simulink model "lab7task"  (R2022b)
settings: Solver=ode45  StartTime=0.0  StopTime=sim_time  RelTol=1e-07  AbsTol=1e-07
values from neighbouring files (symbols this model uses):
  a = 6371+2000    (= 8371)    [lab7taskm.m]
  A0 = [1 0 0; 0 1 0; 0 0 1]    [lab7task1m.m]    (also in lab7taskm.m)
  area = [.06 .06 .04 .06 .06 .04 .12 .12 .12 .12]    [lab7taskm.m]
  C_D = 0.2    [lab7taskm.m]
  density = 0    [lab7taskm.m]
  e = 0.1    [lab7taskm.m]
  eps_Sun = deg2rad(23.45)    [lab7taskm.m]
  euler312_0 = [-atan2(A0(2,1),A0(2,2)); asin(A0(2,3)); -atan2(A0(1,3),A0(3,3))]    [lab7task1m.m]    (also in lab7taskm.m)
  euler313_0 = [-atan2(A0(3,1),A0(3,2)); asin(A0(3,3)); atan2(A0(1,3),A0(2,3))]    [lab7task1m.m]    (also in lab7taskm.m)
  gamma0 = [0;0;1]    [lab7task1m.m]    (also in lab7taskm.m)
  H0 = sqrt((-29615e-9)^2+(-1728e-9)^2+(5186e-9)^2)    [lab7taskm.m]
  I = diag(I)    [lab7task1m.m]    (also in lab7taskm.m)
  I_inv = pinv(I)    [lab7task1m.m]    (also in lab7taskm.m)
  incli = deg2rad(10)    [lab7taskm.m]
  Ir = 0.005    [lab7task1m.m]    (also in lab7taskm.m)
  k = [0;0;1]    [lab7task1m.m]    (also in lab7taskm.m)
  M = [0;0;0]    [lab7task1m.m]    (also in lab7taskm.m)
  m_par = [0.01;0.05;0.01]    [lab7taskm.m]
  mag_tilt = deg2rad(11.5)    [lab7taskm.m]
  Mr = 0    [lab7task1m.m]    (also in lab7taskm.m)
  mu_E = 398600    [lab7task1m.m]    (also in lab7taskm.m = 398600.4418)
  n = sqrt(mu_E/(height+R_E)^3)    [lab7task1m.m]    (also in lab7taskm.m = sqrt(mu_E/a^3))
  n_Sun = sqrt(132712440017.987/R_Sun^3)    [lab7taskm.m]
  Normals = zeros(3,10)    [lab7taskm.m]
  nsurfs = 10    [lab7taskm.m]
  pos = pos-pos_CG    [lab7taskm.m]
  q0 = zeros(4,1)    [lab7task1m.m]    (also in lab7taskm.m)
  R_equat = 6371    [lab7taskm.m]
  R_Sun = 149597870.691    [lab7taskm.m]
  radpressure = radiation/(3e8)    (= 4.52666666667e-06)    [lab7taskm.m]
  rho_d = [.1 .1 .1 .1 .1 .1 .1 .1 .1 .1]    [lab7taskm.m]
  rho_s = [.5 .5 .5 .5 .5 .5 .5 .5 .5 .5]    [lab7taskm.m]
  theta0 = 0    [lab7taskm.m]
  w0 = cat(1,w0,wr0)    [lab7task1m.m]    (also in lab7taskm.m)
  w_E = 2*pi/(23*3600+56*60+4.09)    (= 7.29211590023e-05)    [lab7taskm.m]
libraries: matrix_library x7, vrlib x5
settings Model: Creator=a1pab  LastModifiedBy=a1pab

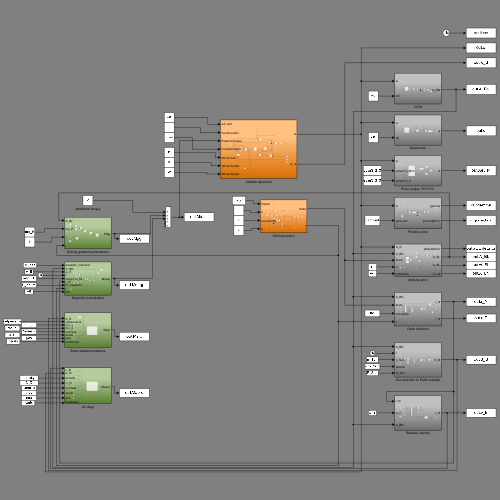
[thumbnail: Simulink's stored preview of the top-level diagram]
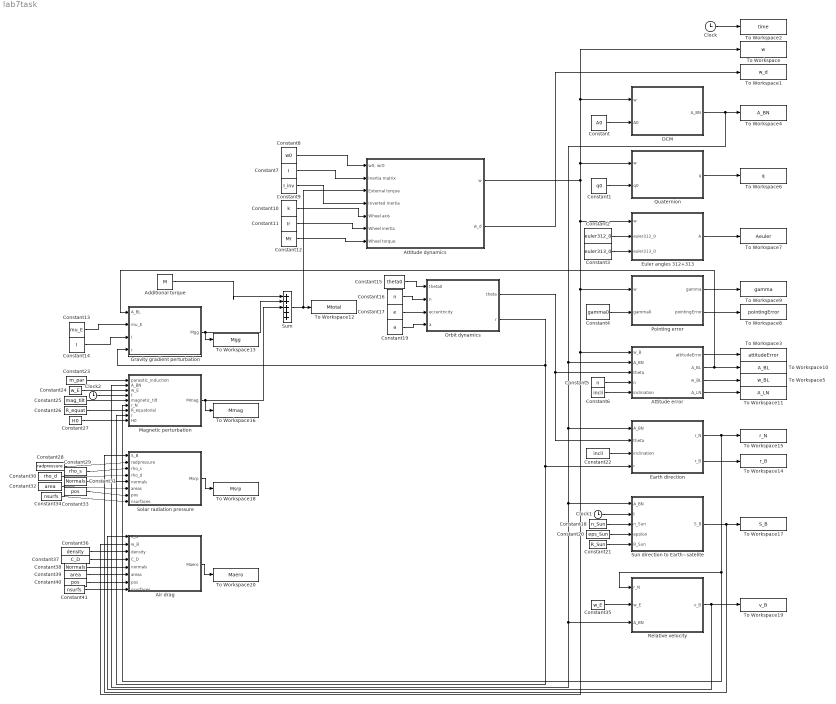
== system lab7task ==
  Additional torque : Constant  Value=M  VectorParams1D=off
  Air drag : Subsystem
  Attitude dynamics : Subsystem
  Attitude error : Subsystem
  Clock : Clock
  Clock1 : Clock
  Clock2 : Clock
  Constant : Constant  Value=A0  VectorParams1D=off
  Constant1 : Constant  Value=q0  VectorParams1D=off
  Constant10 : Constant  Value=k  VectorParams1D=off
  Constant11 : Constant  Value=Ir
  Constant12 : Constant  Value=Mr
  Constant13 : Constant  Value=mu_E
  Constant14 : Constant  Value=I  VectorParams1D=off
  Constant15 : Constant  Value=theta0
  Constant16 : Constant  Value=n
  Constant17 : Constant  Value=e
  Constant18 : Constant  Value=n_Sun
  Constant19 : Constant  Value=a
  Constant2 : Constant  Value=euler312_0  VectorParams1D=off
  Constant20 : Constant  Value=eps_Sun
  Constant21 : Constant  Value=R_Sun
  Constant22 : Constant  Value=incli
  Constant23 : Constant  Value=m_par  VectorParams1D=off
  Constant24 : Constant  Value=w_E
  Constant25 : Constant  Value=mag_tilt
  Constant26 : Constant  Value=R_equat
  Constant27 : Constant  Value=H0
  Constant28 : Constant  Value=radpressure
  Constant29 : Constant  Value=rho_s  VectorParams1D=off
  Constant3 : Constant  Value=euler313_0  VectorParams1D=off
  Constant30 : Constant  Value=rho_d  VectorParams1D=off
  Constant31 : Constant  Value=Normals  VectorParams1D=off
  Constant32 : Constant  Value=area  VectorParams1D=off
  Constant33 : Constant  Value=pos  VectorParams1D=off
  Constant34 : Constant  Value=nsurfs
  Constant35 : Constant  Value=w_E
  Constant36 : Constant  Value=density
  Constant37 : Constant  Value=C_D
  Constant38 : Constant  Value=Normals  VectorParams1D=off
  Constant39 : Constant  Value=area  VectorParams1D=off
  Constant4 : Constant  Value=gamma0  VectorParams1D=off
  Constant40 : Constant  Value=pos  VectorParams1D=off
  Constant41 : Constant  Value=nsurfs
  Constant5 : Constant  Value=n
  Constant6 : Constant  Value=incli
  Constant7 : Constant  Value=I  VectorParams1D=off
  Constant8 : Constant  Value=w0  VectorParams1D=off
  Constant9 : Constant  Value=I_inv  VectorParams1D=off
  DCM : Subsystem
  Earth direction : Subsystem
  "Euler angles 312+313 " : Subsystem
  Gravity gradient perturbation : Subsystem
  Magnetic perturbation : Subsystem
  Orbit dynamics : Subsystem
  Pointing error : Subsystem
  Quaternion : Subsystem
  Relative velocity : Subsystem
  Solar radiation pressure : Subsystem
  Sum : Sum  Inputs=|+++++
  Sun direction to Earth~satelite : Subsystem
  To Workspace : ToWorkspace  VariableName=w  SampleTime=-1
  To Workspace1 : ToWorkspace  VariableName=w_d  SampleTime=-1
  To Workspace10 : ToWorkspace  VariableName=A_BL  SampleTime=-1
  To Workspace11 : ToWorkspace  VariableName=A_LN  SampleTime=-1
  To Workspace12 : ToWorkspace  VariableName=Mtotal  SampleTime=-1
  To Workspace13 : ToWorkspace  VariableName=Mgg  SampleTime=-1
  To Workspace14 : ToWorkspace  VariableName=r_B  SampleTime=-1
  To Workspace15 : ToWorkspace  VariableName=r_N  SampleTime=-1
  To Workspace16 : ToWorkspace  VariableName=Mmag  SampleTime=-1
  To Workspace17 : ToWorkspace  VariableName=S_B  SampleTime=-1
  To Workspace18 : ToWorkspace  VariableName=Msrp  SampleTime=-1
  To Workspace19 : ToWorkspace  VariableName=v_B  SampleTime=-1
  To Workspace2 : ToWorkspace  VariableName=time  SampleTime=-1
  To Workspace20 : ToWorkspace  VariableName=Maero  SampleTime=-1
  To Workspace3 : ToWorkspace  VariableName=attitudeError  SampleTime=-1
  To Workspace4 : ToWorkspace  VariableName=A_BN  SampleTime=-1
  To Workspace5 : ToWorkspace  VariableName=w_BL  SampleTime=-1
  To Workspace6 : ToWorkspace  VariableName=q  SampleTime=-1
  To Workspace7 : ToWorkspace  VariableName=Aeuler  SampleTime=-1
  To Workspace8 : ToWorkspace  VariableName=pointingError  SampleTime=-1
  To Workspace9 : ToWorkspace  VariableName=gamma  SampleTime=-1
  wires:
  Attitude dynamics/1(w) -> Air drag/2(w_B), Attitude error/1(w_B), Pointing error/1(w), "Euler angles 312+313 "/1(w), Quaternion/1(w), To Workspace/1, DCM/1(w)
  Attitude dynamics/2(w_d) -> To Workspace1/1
  Clock/1 -> To Workspace2/1
  Constant10/1 -> Attitude dynamics/5(Wheel axis)
  Constant11/1 -> Attitude dynamics/6(Wheel inertia)
  Constant12/1 -> Attitude dynamics/7(Wheel torque)
  Constant8/1 -> Attitude dynamics/1("w0, wr0")
  Constant7/1 -> Attitude dynamics/2(Inertia matrix)
  Constant9/1 -> Attitude dynamics/4(Inverted Inertia)
  Constant/1 -> DCM/2(A0)
  Constant1/1 -> Quaternion/2(q0)
  Quaternion/1(q) -> To Workspace6/1
  Constant2/1 -> "Euler angles 312+313 "/2(euler312_0)
  Constant3/1 -> "Euler angles 312+313 "/3(euler313_0)
  "Euler angles 312+313 "/1(A) -> To Workspace7/1
  Constant4/1 -> Pointing error/2(gamma0)
  Pointing error/2(pointingError) -> To Workspace8/1
  Pointing error/1(gamma) -> To Workspace9/1
  Attitude error/1(attitudeError) -> To Workspace3/1
  Attitude error/3(w_BL) -> To Workspace5/1
  Orbit dynamics/1(theta) -> Earth direction/2(theta), Attitude error/3(theta)
  Constant5/1 -> Attitude error/4(n)
  Additional torque/1 -> Sum/1
  Gravity gradient perturbation/1(Mgg) -> Sum/2, To Workspace13/1
  Sum/1 -> Attitude dynamics/3(External torque), To Workspace12/1
  Attitude error/2(A_BL) -> To Workspace10/1, Gravity gradient perturbation/1(A_BL)
  Constant13/1 -> Gravity gradient perturbation/2(mu_E)
  Constant14/1 -> Gravity gradient perturbation/3(I)
  Attitude error/4(A_LN) -> To Workspace11/1
  Constant6/1 -> Attitude error/5(inclination)
  Constant15/1 -> Orbit dynamics/1(theta0)
  Constant16/1 -> Orbit dynamics/2(n)
  Constant17/1 -> Orbit dynamics/3(eccentricity)
  Constant19/1 -> Orbit dynamics/4(a)
  Orbit dynamics/2(r) -> Gravity gradient perturbation/4(r), Magnetic perturbation/8(r), Earth direction/4(r)
  DCM/1(A_BN) -> Sun direction to Earth~satelite/1(A_BN), Magnetic perturbation/2(A_BN), Relative velocity/3(A_BN), Earth direction/1(A_BN), Attitude error/2(A_BN), To Workspace4/1
  Constant20/1 -> Sun direction to Earth~satelite/4(epsilon)
  Constant18/1 -> Sun direction to Earth~satelite/3(n_Sun)
  Constant22/1 -> Earth direction/3(inclination)
  Clock1/1 -> Sun direction to Earth~satelite/2(t)
  Earth direction/2(r_B) -> To Workspace14/1
  Earth direction/1(r_N) -> Relative velocity/1(r_N), Magnetic perturbation/6(r_N), To Workspace15/1
  Sun direction to Earth~satelite/1(S_B) -> Solar radiation pressure/1(S_B), To Workspace17/1
  Constant21/1 -> Sun direction to Earth~satelite/5(R_Sun)
  Magnetic perturbation/1(Mmag) -> Sum/3, To Workspace16/1
  Constant23/1 -> Magnetic perturbation/1(parasitic_induction)
  Constant24/1 -> Magnetic perturbation/3(w_E)
  Clock2/1 -> Magnetic perturbation/4(t)
  Constant25/1 -> Magnetic perturbation/5(magnetic_tilt)
  Constant26/1 -> Magnetic perturbation/7(R_equatorial)
  Constant27/1 -> Magnetic perturbation/9(H0)
  Solar radiation pressure/1(Msrp) -> To Workspace18/1
  Constant28/1 -> Solar radiation pressure/2(radpressure)
  Constant29/1 -> Solar radiation pressure/3(rho_s)
  Constant30/1 -> Solar radiation pressure/4(rho_d)
  Constant31/1 -> Solar radiation pressure/5(normals)
  Constant32/1 -> Solar radiation pressure/6(areas)
  Constant33/1 -> Solar radiation pressure/7(pos)
  Constant34/1 -> Solar radiation pressure/8(nsurfaces)
  Constant35/1 -> Relative velocity/2(w_E)
  Relative velocity/1(v_B) -> Air drag/1(v_B), To Workspace19/1
  Air drag/1(Maero) -> To Workspace20/1
  Constant36/1 -> Air drag/3(density)
  Constant37/1 -> Air drag/4(C_D)
  Constant38/1 -> Air drag/5(normals)
  Constant39/1 -> Air drag/6(areas)
  Constant40/1 -> Air drag/7(pos)
  Constant41/1 -> Air drag/8(nsurfaces)

== system lab7task/Air drag ==
  v_B : Inport
  w_B : Inport  Port=2
  density : Inport  Port=3
  C_D : Inport  Port=4
  normals : Inport  Port=5
  areas : Inport  Port=6
  pos : Inport  Port=7
  nsurfaces : Inport  Port=8
  For Iterator Subsystem : Subsystem  TreatAsAtomicUnit=on
  Maero : Outport
  wires:
  normals/1 -> For Iterator Subsystem/5(normals)
  areas/1 -> For Iterator Subsystem/6(areas)
  pos/1 -> For Iterator Subsystem/7(pos)
  nsurfaces/1 -> For Iterator Subsystem/8(nsurfaces)
  For Iterator Subsystem/1(torque) -> Maero/1
  density/1 -> For Iterator Subsystem/3(density)
  v_B/1 -> For Iterator Subsystem/1(v_B)
  w_B/1 -> For Iterator Subsystem/2(w_B)
  C_D/1 -> For Iterator Subsystem/4(C_D)

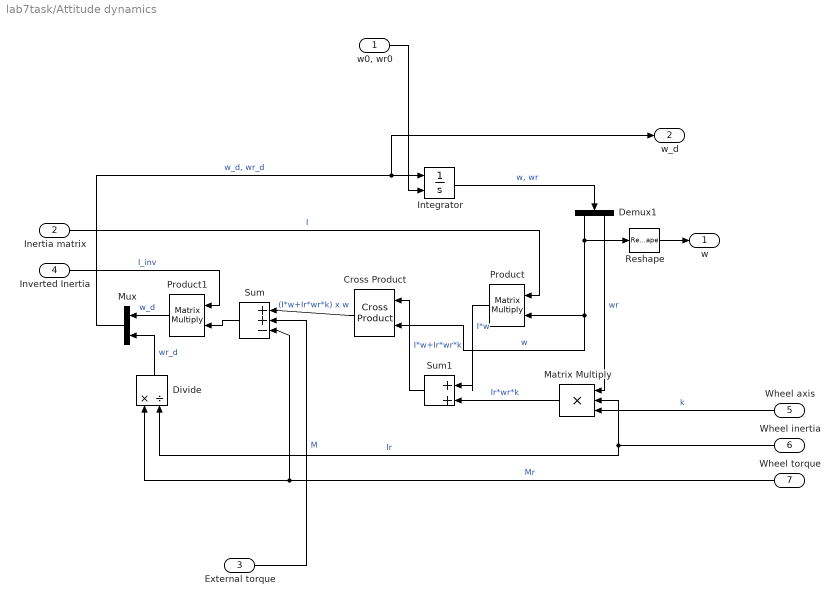
== system lab7task/Attitude dynamics ==
  "w0, wr0" : Inport
  Inertia matrix : Inport  Port=2
  External torque : Inport  Port=3
  Inverted Inertia : Inport  Port=4
  Wheel axis : Inport  Port=5
  Wheel inertia : Inport  Port=6
  Wheel torque : Inport  Port=7
  Cross Product : matrix_library/Cross Product
  Demux1 : Demux  Outputs=2
  Divide : Product  Inputs=*/
  Integrator : Integrator  InitialConditionSource=external
  Matrix Multiply : Product  Inputs=3
  Mux : Mux  Inputs=2
  Product : Product  Multiplication=Matrix(*)
  Product1 : Product  Multiplication=Matrix(*)
  Reshape : Reshape  OutputDimensionality=Column vector (2-D)
  Sum : Sum  Inputs=|++-
  Sum1 : Sum  Inputs=|++
  w : Outport
  w_d : Outport  Port=2
  wires:
  Mux/1 -> w_d/1, Integrator/1  "w_d, wr_d"
  Integrator/1 -> Demux1/1  "w, wr"
  "w0, wr0"/1 -> Integrator/2
  Product/1 -> Sum1/1  "I*w"
  Cross Product/1 -> Sum/1  "(I*w+Ir*wr*k) x w"
  Inertia matrix/1 -> Product/1  "I"
  External torque/1 -> Sum/2  "M"
  Product1/1 -> Mux/1  "w_d"
  Wheel torque/1 -> Sum/3, Divide/1  "Mr"
  Wheel inertia/1 -> Divide/2, Matrix Multiply/2  "Ir"
  Divide/1 -> Mux/2  "wr_d"
  Demux1/1 -> Reshape/1, Cross Product/2, Product/2  "w"
  Sum1/1 -> Cross Product/1  "I*w+Ir*wr*k"
  Demux1/2 -> Matrix Multiply/1  "wr"
  Matrix Multiply/1 -> Sum1/2  "Ir*wr*k"
  Wheel axis/1 -> Matrix Multiply/3  "k"
  Reshape/1 -> w/1
  Sum/1 -> Product1/2
  Inverted Inertia/1 -> Product1/1  "I_inv"

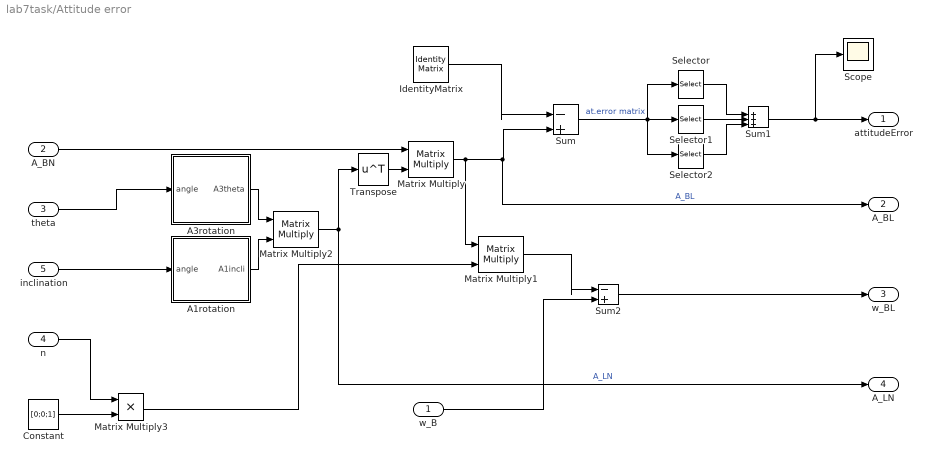
== system lab7task/Attitude error ==
  w_B : Inport
  A_BN : Inport  Port=2
  theta : Inport  Port=3
  n : Inport  Port=4
  inclination : Inport  Port=5
  A1rotation : Subsystem
  A3rotation : Subsystem
  Constant : Constant  Value=[0;0;1]  VectorParams1D=off
  IdentityMatrix : IdentityMatrix  OutputDimensions=3
  Matrix Multiply : Product  Multiplication=Matrix(*)
  Matrix Multiply1 : Product  Multiplication=Matrix(*)
  Matrix Multiply2 : Product  Multiplication=Matrix(*)
  Matrix Multiply3 : Product
  Scope : Scope
  Selector : Selector  NumberOfDimensions=2  InputPortWidth=3  IndexOptions=Index vector (dialog),Index vector (dialog)  Indices=1,1  OutputSizes=1,1
  Selector1 : Selector  NumberOfDimensions=2  InputPortWidth=3  IndexOptions=Index vector (dialog),Index vector (dialog)  Indices=2,2  OutputSizes=1,1
  Selector2 : Selector  NumberOfDimensions=2  InputPortWidth=3  IndexOptions=Index vector (dialog),Index vector (dialog)  Indices=3,3  OutputSizes=1,1
  Sum : Sum  Inputs=|-+
  Sum1 : Sum  Inputs=|+++
  Sum2 : Sum  Inputs=|-+
  Transpose : Math  Operator=transpose
  attitudeError : Outport
  A_BL : Outport  Port=2
  w_BL : Outport  Port=3
  A_LN : Outport  Port=4
  wires:
  n/1 -> Matrix Multiply3/1
  theta/1 -> A3rotation/1(angle)
  Transpose/1 -> Matrix Multiply/2
  A_BN/1 -> Matrix Multiply/1
  Matrix Multiply/1 -> Matrix Multiply1/1, A_BL/1, Sum/2  "A_BL"
  IdentityMatrix/1 -> Sum/1
  Sum/1 -> Selector/1, Selector1/1, Selector2/1  "at.error matrix"
  Selector/1 -> Sum1/1
  Selector1/1 -> Sum1/2
  Selector2/1 -> Sum1/3
  w_B/1 -> Sum2/2
  Matrix Multiply1/1 -> Sum2/1
  Sum1/1 -> Scope/1, attitudeError/1
  Sum2/1 -> w_BL/1
  Constant/1 -> Matrix Multiply3/2
  Matrix Multiply3/1 -> Matrix Multiply1/2
  inclination/1 -> A1rotation/1(angle)
  A3rotation/1(A3theta) -> Matrix Multiply2/1
  A1rotation/1(A1incli) -> Matrix Multiply2/2
  Matrix Multiply2/1 -> A_LN/1, Transpose/1  "A_LN"

== system lab7task/DCM ==
  w : Inport
  A0 : Inport  Port=2
  3x3 Skew-symmetric matrix : Subsystem
  Integrator : Integrator  InitialConditionSource=external
  Matrix Multiply : Product  Multiplication=Matrix(*)
  Matrix Multiply1 : Product  Multiplication=Matrix(*)
  Matrix Multiply2 : Product  Multiplication=Matrix(*)
  Multiply : Gain  Gain=-1
  Multiply1 : Gain  Gain=1.5
  Multiply2 : Gain  Gain=0.5
  Sum : Sum  Inputs=|+-
  Transpose : Math  Operator=transpose
  A_BN : Outport
  wires:
  w/1 -> 3x3 Skew-symmetric matrix/1(w)
  3x3 Skew-symmetric matrix/1(w^) -> Multiply/1
  Multiply/1 -> Matrix Multiply/1
  Matrix Multiply/1 -> Integrator/1
  A0/1 -> Integrator/2
  Integrator/1 -> Transpose/1, Matrix Multiply2/2, Multiply2/1, Multiply1/1
  Transpose/1 -> Matrix Multiply1/2
  Sum/1 -> Matrix Multiply/2, A_BN/1
  Matrix Multiply1/1 -> Matrix Multiply2/1
  Matrix Multiply2/1 -> Sum/2
  Multiply1/1 -> Sum/1
  Multiply2/1 -> Matrix Multiply1/1

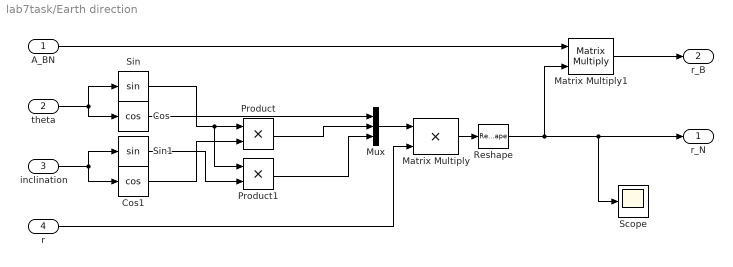
== system lab7task/Earth direction ==
  A_BN : Inport
  theta : Inport  Port=2
  inclination : Inport  Port=3
  r : Inport  Port=4
  Cos : Trigonometry  Operator=cos
  Cos1 : Trigonometry  Operator=cos
  Matrix Multiply : Product
  Matrix Multiply1 : Product  Multiplication=Matrix(*)
  Mux : Mux  Inputs=3
  Product : Product
  Product1 : Product
  Reshape : Reshape  OutputDimensionality=Column vector (2-D)
  Scope : Scope
  Sin : Trigonometry
  Sin1 : Trigonometry
  r_N : Outport
  r_B : Outport  Port=2
  wires:
  theta/1 -> Cos/1, Sin/1
  inclination/1 -> Sin1/1, Cos1/1
  Cos/1 -> Mux/1
  Mux/1 -> Matrix Multiply/1
  r/1 -> Matrix Multiply/2
  Sin/1 -> Product1/1, Product/1
  Cos1/1 -> Product/2
  Sin1/1 -> Product1/2
  Product/1 -> Mux/2
  Product1/1 -> Mux/3
  Matrix Multiply/1 -> Reshape/1
  Reshape/1 -> Scope/1, r_N/1, Matrix Multiply1/2
  A_BN/1 -> Matrix Multiply1/1
  Matrix Multiply1/1 -> r_B/1

== system lab7task/Euler angles 312+313  ==
  w : Inport
  euler312_0 : Inport  Port=2
  euler313_0 : Inport  Port=3
  Abs : Abs  SaturateOnIntegerOverflow=off
  If : If  IfExpression=u1 > 0.1
  If Action Subsystem : Subsystem  TreatAsAtomicUnit=on
  If Action Subsystem1 : Subsystem  TreatAsAtomicUnit=on
  Integrate euler312 : Subsystem
  Integrate euler313 : Subsystem
  Switch : Switch  Criteria=u2 > Threshold  Threshold=0.1  SaturateOnIntegerOverflow=off  InputSameDT=off
  A : Outport
  wires:
  w/1 -> Integrate euler313/1(w), Integrate euler312/1(w)
  euler312_0/1 -> Integrate euler312/2(angles0)
  euler313_0/1 -> Integrate euler313/2(angles0)
  Integrate euler312/2(cos(theta)312) -> Abs/1
  Abs/1 -> Switch/2, If/1
  Integrate euler312/1(euler312) -> If Action Subsystem/1(euler312)
  If/1 -> If Action Subsystem/Action
  Integrate euler313/1(euler313) -> If Action Subsystem1/1(euler313)
  If/2 -> If Action Subsystem1/Action
  If Action Subsystem/1(A) -> Switch/1
  If Action Subsystem1/1(A) -> Switch/3
  Switch/1 -> A/1

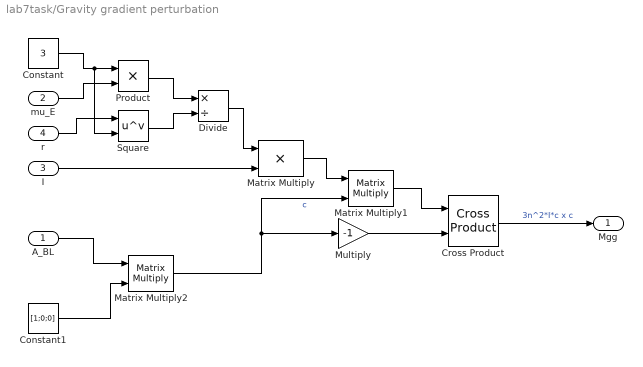
== system lab7task/Gravity gradient perturbation ==
  A_BL : Inport
  mu_E : Inport  Port=2
  I : Inport  Port=3
  r : Inport  Port=4
  Constant : Constant  Value=3
  Constant1 : Constant  Value=[1;0;0]  VectorParams1D=off
  Cross Product : matrix_library/Cross Product
  Divide : Product  Inputs=*/
  Matrix Multiply : Product
  Matrix Multiply1 : Product  Multiplication=Matrix(*)
  Matrix Multiply2 : Product  Multiplication=Matrix(*)
  Multiply : Gain  Gain=-1
  Product : Product
  Square : Math  Operator=pow
  Mgg : Outport
  wires:
  Constant/1 -> Square/2, Product/1
  mu_E/1 -> Product/2
  I/1 -> Matrix Multiply/2
  Matrix Multiply/1 -> Matrix Multiply1/1
  Matrix Multiply1/1 -> Cross Product/1
  Cross Product/1 -> Mgg/1  "3n^2*I*c x c"
  A_BL/1 -> Matrix Multiply2/1
  Constant1/1 -> Matrix Multiply2/2
  Matrix Multiply2/1 -> Multiply/1, Matrix Multiply1/2  "c"
  Divide/1 -> Matrix Multiply/1
  Product/1 -> Divide/1
  Square/1 -> Divide/2
  r/1 -> Square/1
  Multiply/1 -> Cross Product/2

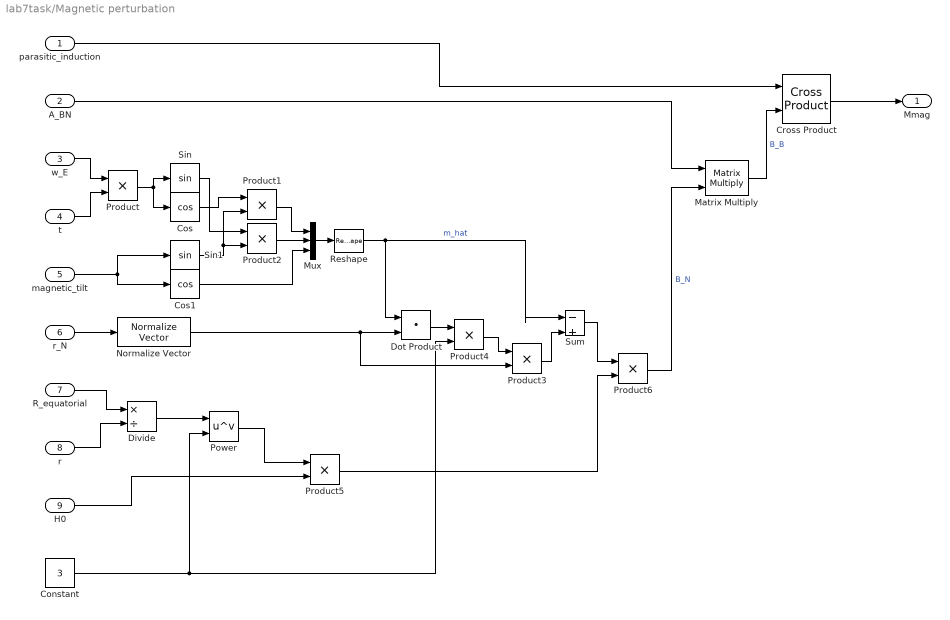
== system lab7task/Magnetic perturbation ==
  parasitic_induction : Inport
  A_BN : Inport  Port=2
  w_E : Inport  Port=3
  t : Inport  Port=4
  magnetic_tilt : Inport  Port=5
  r_N : Inport  Port=6
  R_equatorial : Inport  Port=7
  r : Inport  Port=8
  H0 : Inport  Port=9
  Constant : Constant  Value=3
  Cos : Trigonometry  Operator=cos
  Cos1 : Trigonometry  Operator=cos
  Cross Product : matrix_library/Cross Product
  Divide : Product  Inputs=*/
  Dot Product : DotProduct  OutDataTypeStr=Inherit: Inherit via internal rule
  Matrix Multiply : Product  Multiplication=Matrix(*)
  Mux : Mux  Inputs=3
  Normalize Vector : vrlib/Utilities/Normalize Vector  maxzero=0
  Power : Math  Operator=pow
  Product{,1..6} (7 alike) : Product
  Reshape : Reshape  OutputDimensionality=Column vector (2-D)
  Sin : Trigonometry
  Sin1 : Trigonometry
  Sum : Sum  Inputs=|-+
  Mmag : Outport
  wires:
  w_E/1 -> Product/1
  t/1 -> Product/2
  magnetic_tilt/1 -> Sin1/1, Cos1/1
  Product/1 -> Cos/1, Sin/1
  Cos/1 -> Product1/1
  Sin1/1 -> Product2/2, Product1/2
  Sin/1 -> Product2/1
  Product2/1 -> Mux/2
  Product1/1 -> Mux/1
  Cos1/1 -> Mux/3
  Mux/1 -> Reshape/1
  Reshape/1 -> Dot Product/1, Sum/1  "m_hat"
  r_N/1 -> Normalize Vector/1
  Normalize Vector/1 -> Product3/2, Dot Product/2
  Product3/1 -> Sum/2
  Dot Product/1 -> Product4/1
  Constant/1 -> Power/2, Product4/2
  Product4/1 -> Product3/1
  R_equatorial/1 -> Divide/1
  r/1 -> Divide/2
  Divide/1 -> Power/1
  Power/1 -> Product5/1
  H0/1 -> Product5/2
  Sum/1 -> Product6/1
  Product5/1 -> Product6/2
  Product6/1 -> Matrix Multiply/2  "B_N"
  A_BN/1 -> Matrix Multiply/1
  parasitic_induction/1 -> Cross Product/1
  Matrix Multiply/1 -> Cross Product/2  "B_B"
  Cross Product/1 -> Mmag/1

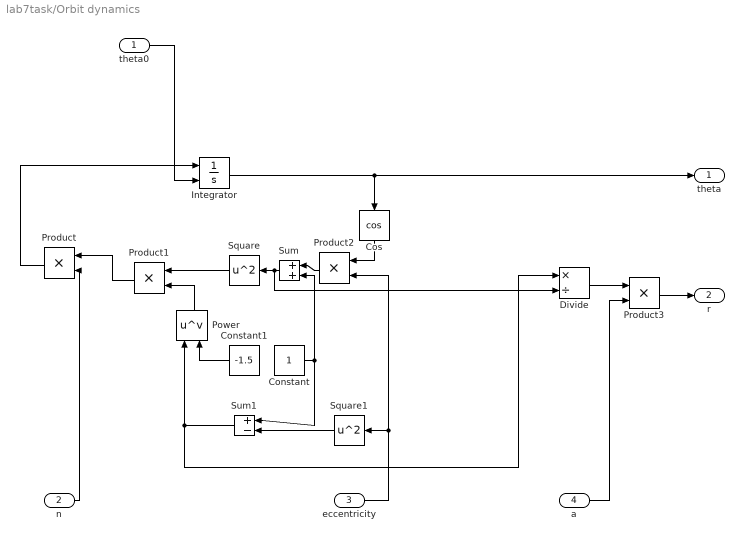
== system lab7task/Orbit dynamics ==
  theta0 : Inport
  n : Inport  Port=2
  eccentricity : Inport  Port=3
  a : Inport  Port=4
  Constant : Constant
  Constant1 : Constant  Value=-1.5
  Cos : Trigonometry  Operator=cos
  Divide : Product  Inputs=*/
  Integrator : Integrator  InitialConditionSource=external
  Power : Math  Operator=pow
  Product{,1..3} (4 alike) : Product
  Square : Math  Operator=square
  Square1 : Math  Operator=square
  Sum : Sum  Inputs=|++
  Sum1 : Sum  Inputs=|+-
  theta : Outport
  r : Outport  Port=2
  wires:
  theta0/1 -> Integrator/2
  Integrator/1 -> Cos/1, theta/1
  Product/1 -> Integrator/1
  Cos/1 -> Product2/1
  eccentricity/1 -> Product2/2, Square1/1
  Product2/1 -> Sum/1
  Constant/1 -> Sum1/1, Sum/2
  n/1 -> Product/2
  Sum/1 -> Divide/2, Square/1
  Square/1 -> Product1/1
  Product1/1 -> Product/1
  Power/1 -> Product1/2
  Constant1/1 -> Power/2
  Square1/1 -> Sum1/2
  Sum1/1 -> Divide/1, Power/1
  Divide/1 -> Product3/1
  a/1 -> Product3/2
  Product3/1 -> r/1

== system lab7task/Pointing error ==
  w : Inport
  gamma0 : Inport  Port=2
  Acos : Trigonometry  Operator=acos
  Cross Product : matrix_library/Cross Product
  Dot Product : DotProduct  OutDataTypeStr=Inherit: Inherit via internal rule
  Integrator : Integrator  InitialConditionSource=external
  Normalize Vector : vrlib/Utilities/Normalize Vector  maxzero=0
  gamma : Outport
  pointingError : Outport  Port=2
  wires:
  gamma0/1 -> Dot Product/1, Integrator/2
  w/1 -> Cross Product/2
  Cross Product/1 -> Integrator/1
  Integrator/1 -> Normalize Vector/1
  Normalize Vector/1 -> Dot Product/2, gamma/1, Cross Product/1
  Dot Product/1 -> Acos/1
  Acos/1 -> pointingError/1

== system lab7task/Quaternion ==
  w : Inport
  q0 : Inport  Port=2
  4x4 Skew-symmetric matrix : Subsystem
  Integrator : Integrator  InitialConditionSource=external
  Matrix Multiply : Product  Multiplication=Matrix(*)
  Multiply : Gain  Gain=0.5
  Normalize Vector : vrlib/Utilities/Normalize Vector  maxzero=0
  q : Outport
  wires:
  w/1 -> 4x4 Skew-symmetric matrix/1(w)
  4x4 Skew-symmetric matrix/1(w^) -> Multiply/1
  Multiply/1 -> Matrix Multiply/1
  Matrix Multiply/1 -> Integrator/1
  q0/1 -> Integrator/2
  Integrator/1 -> Normalize Vector/1
  Normalize Vector/1 -> Matrix Multiply/2, q/1

== system lab7task/Relative velocity ==
  r_N : Inport
  w_E : Inport  Port=2
  A_BN : Inport  Port=3
  Demux : Demux  Outputs=3
  Derivative : Derivative
  Derivative1 : Derivative
  Derivative2 : Derivative
  Matrix Multiply : Product  Multiplication=Matrix(*)
  Mux : Mux  Inputs=3
  Product : Product
  Product1 : Product
  Sum : Sum  Inputs=|++
  Sum1 : Sum  Inputs=|+-
  v_B : Outport
  wires:
  r_N/1 -> Demux/1
  Demux/3 -> Derivative2/1
  Derivative2/1 -> Mux/3
  Sum/1 -> Mux/1
  Sum1/1 -> Mux/2
  Derivative/1 -> Sum/1
  Derivative1/1 -> Sum1/1
  w_E/1 -> Product/2, Product1/2
  Demux/2 -> Derivative1/1, Product/1
  Demux/1 -> Derivative/1, Product1/1
  Product/1 -> Sum/2
  Product1/1 -> Sum1/2
  A_BN/1 -> Matrix Multiply/1
  Mux/1 -> Matrix Multiply/2  "relative orbit v_N"
  Matrix Multiply/1 -> v_B/1  "rel. orbit v_B"

== system lab7task/Solar radiation pressure ==
  S_B : Inport
  radpressure : Inport  Port=2
  rho_s : Inport  Port=3
  rho_d : Inport  Port=4
  normals : Inport  Port=5
  areas : Inport  Port=6
  pos : Inport  Port=7
  nsurfaces : Inport  Port=8
  For Iterator Subsystem : Subsystem  TreatAsAtomicUnit=on
  Normalize Vector : vrlib/Utilities/Normalize Vector  maxzero=0
  Msrp : Outport
  wires:
  S_B/1 -> Normalize Vector/1
  Normalize Vector/1 -> For Iterator Subsystem/1(S_B)
  radpressure/1 -> For Iterator Subsystem/2(radpressure)
  rho_s/1 -> For Iterator Subsystem/3(rho_s)
  rho_d/1 -> For Iterator Subsystem/4(rho_d)
  normals/1 -> For Iterator Subsystem/5(normals)
  areas/1 -> For Iterator Subsystem/6(areas)
  pos/1 -> For Iterator Subsystem/7(pos)
  nsurfaces/1 -> For Iterator Subsystem/8(nsurfaces)
  For Iterator Subsystem/1(torque) -> Msrp/1

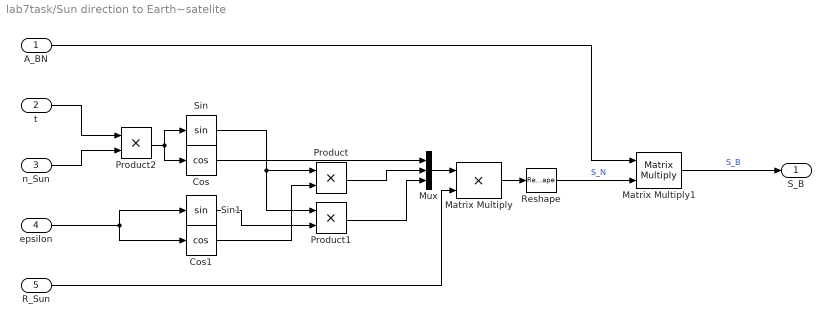
== system lab7task/Sun direction to Earth~satelite ==
  A_BN : Inport
  t : Inport  Port=2
  n_Sun : Inport  Port=3
  epsilon : Inport  Port=4
  R_Sun : Inport  Port=5
  Cos : Trigonometry  Operator=cos
  Cos1 : Trigonometry  Operator=cos
  Matrix Multiply : Product
  Matrix Multiply1 : Product  Multiplication=Matrix(*)
  Mux : Mux  Inputs=3
  Product : Product
  Product1 : Product
  Product2 : Product
  Reshape : Reshape  OutputDimensionality=Column vector (2-D)
  Sin : Trigonometry
  Sin1 : Trigonometry
  S_B : Outport
  wires:
  t/1 -> Product2/1
  n_Sun/1 -> Product2/2
  Product2/1 -> Cos/1, Sin/1
  epsilon/1 -> Cos1/1, Sin1/1
  Cos/1 -> Mux/1
  Sin/1 -> Product1/1, Product/1
  Cos1/1 -> Product/2
  Sin1/1 -> Product1/2
  Product/1 -> Mux/2
  Product1/1 -> Mux/3
  Mux/1 -> Matrix Multiply/1
  Matrix Multiply/1 -> Reshape/1
  R_Sun/1 -> Matrix Multiply/2
  Reshape/1 -> Matrix Multiply1/2  "S_N"
  A_BN/1 -> Matrix Multiply1/1
  Matrix Multiply1/1 -> S_B/1  "S_B"

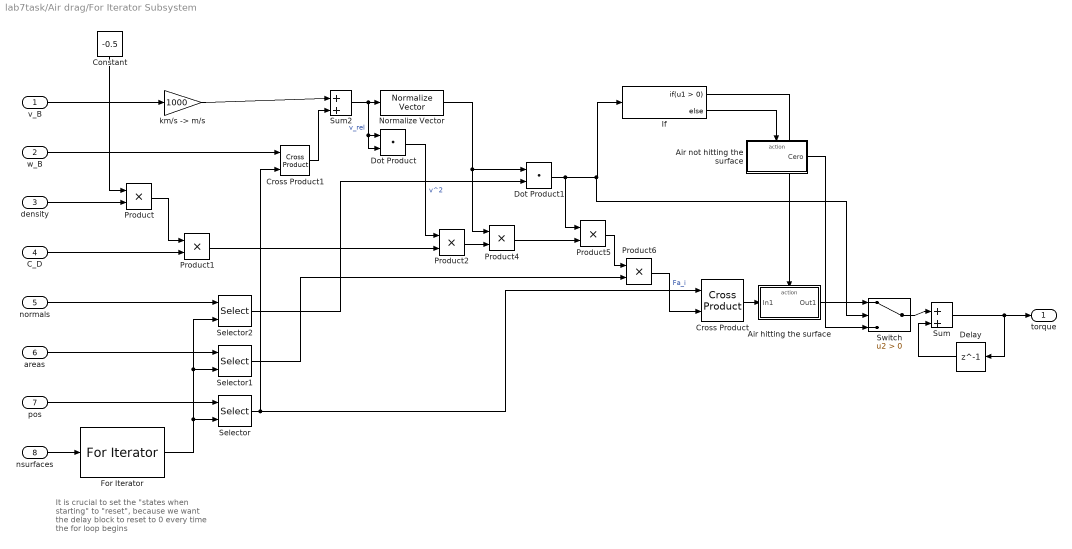
== system lab7task/Air drag/For Iterator Subsystem ==
  note: It is crucial to set the "states when
      | starting" to "reset", because we want
      | the delay block to reset to 0 every
      | time the for loop begins
  v_B : Inport
  w_B : Inport  Port=2
  density : Inport  Port=3
  C_D : Inport  Port=4
  normals : Inport  Port=5
  areas : Inport  Port=6
  pos : Inport  Port=7
  nsurfaces : Inport  Port=8
  Air hitting the surface : Subsystem  TreatAsAtomicUnit=on
  Air not hitting the surface : Subsystem  TreatAsAtomicUnit=on
  Constant : Constant  Value=-0.5
  Cross Product : matrix_library/Cross Product
  Cross Product1 : matrix_library/Cross Product
  Delay : Delay  DelayLength=1
  Dot Product : DotProduct  OutDataTypeStr=Inherit: Inherit via internal rule
  Dot Product1 : DotProduct  OutDataTypeStr=Inherit: Inherit via internal rule
  For Iterator : ForIterator  ResetStates=reset  IterationSource=external
  If : If
  Normalize Vector : vrlib/Utilities/Normalize Vector  maxzero=0
  Product{,1..2,4..6} (6 alike) : Product
  Selector : Selector  NumberOfDimensions=2  InputPortWidth=3  IndexOptions=Select all,Index vector (port)  Indices=[1 3],1  OutputSizes=1,1
  Selector1 : Selector  NumberOfDimensions=2  InputPortWidth=3  IndexOptions=Select all,Index vector (port)  Indices=[1 3],1  OutputSizes=1,1
  Selector2 : Selector  NumberOfDimensions=2  InputPortWidth=3  IndexOptions=Select all,Index vector (port)  Indices=[1 3],1  OutputSizes=1,1
  Sum : Sum  Inputs=|++
  Sum2 : Sum  Inputs=|++
  Switch : Switch  Criteria=u2 > Threshold  SaturateOnIntegerOverflow=off  InputSameDT=off
  "km/s -> m/s" : Gain  Gain=1000
  torque : Outport
  wires:
  nsurfaces/1 -> For Iterator/1
  Delay/1 -> Sum/2
  Sum/1 -> torque/1, Delay/1
  For Iterator/1 -> Selector1/2, Selector2/2, Selector/2
  pos/1 -> Selector/1
  normals/1 -> Selector2/1
  areas/1 -> Selector1/1
  Air not hitting the surface/1(Cero) -> Switch/3
  If/1 -> Air hitting the surface/Action
  If/2 -> Air not hitting the surface/Action
  Switch/1 -> Sum/1
  Air hitting the surface/1(Out1) -> Switch/1
  Cross Product/1 -> Air hitting the surface/1(In1)
  v_B/1 -> "km/s -> m/s"/1
  w_B/1 -> Cross Product1/1
  Selector/1 -> Cross Product/1, Cross Product1/2
  Cross Product1/1 -> Sum2/2
  Sum2/1 -> Dot Product/2, Dot Product/1, Normalize Vector/1  "v_rel"
  Dot Product/1 -> Product2/1  "v^2"
  density/1 -> Product/2
  Constant/1 -> Product/1
  C_D/1 -> Product1/2
  Product/1 -> Product1/1
  Product1/1 -> Product2/2
  Product2/1 -> Product4/2
  Normalize Vector/1 -> Product4/1, Dot Product1/1
  Dot Product1/1 -> Product5/1, Switch/2, If/1
  Selector2/1 -> Dot Product1/2
  Product4/1 -> Product5/2
  Product5/1 -> Product6/1
  Selector1/1 -> Product6/2
  Product6/1 -> Cross Product/2  "Fa_i"
  "km/s -> m/s"/1 -> Sum2/1

== system lab7task/Attitude error/A1rotation ==
  angle : Inport
  Constant : Constant
  Constant1 : Constant  Value=0
  Cos : Trigonometry  Operator=cos
  Display : Display
  Matrix Concatenate : Concatenate  NumInputs=3  Mode=Multidimensional array  ConcatenateDimension=2
  Multiply : Gain  Gain=-1
  Selector : Selector  InputPortWidth=5  IndexOptions=Index vector (dialog)  Indices=[1 2 2]  OutputSizes=1
  Selector1 : Selector  InputPortWidth=5  IndexOptions=Index vector (dialog)  Indices=[2 5 4]  OutputSizes=1
  Selector2 : Selector  InputPortWidth=5  IndexOptions=Index vector (dialog)  Indices=[2 3 5]  OutputSizes=1
  Sin : Trigonometry
  Vector Concatenate : Concatenate  NumInputs=5
  A1incli : Outport
  wires:
  angle/1 -> Cos/1, Sin/1
  Sin/1 -> Vector Concatenate/3, Multiply/1
  Constant/1 -> Vector Concatenate/1
  Constant1/1 -> Vector Concatenate/2
  Multiply/1 -> Vector Concatenate/4
  Cos/1 -> Vector Concatenate/5
  Vector Concatenate/1 -> Selector2/1, Selector1/1, Selector/1
  Selector/1 -> Matrix Concatenate/1
  Selector1/1 -> Matrix Concatenate/2
  Selector2/1 -> Matrix Concatenate/3
  Matrix Concatenate/1 -> Display/1, A1incli/1

== system lab7task/Attitude error/A3rotation ==
  angle : Inport
  Constant : Constant
  Constant1 : Constant  Value=0
  Cos : Trigonometry  Operator=cos
  Display : Display
  Matrix Concatenate : Concatenate  NumInputs=3  Mode=Multidimensional array  ConcatenateDimension=2
  Multiply : Gain  Gain=-1
  Selector : Selector  InputPortWidth=5  IndexOptions=Index vector (dialog)  Indices=[5 4 2]  OutputSizes=1
  Selector1 : Selector  InputPortWidth=5  IndexOptions=Index vector (dialog)  Indices=[3 5 2]  OutputSizes=1
  Selector2 : Selector  InputPortWidth=5  IndexOptions=Index vector (dialog)  Indices=[2 2 1]  OutputSizes=1
  Sin : Trigonometry
  Vector Concatenate : Concatenate  NumInputs=5
  A3theta : Outport
  wires:
  angle/1 -> Cos/1, Sin/1
  Sin/1 -> Vector Concatenate/3, Multiply/1
  Constant/1 -> Vector Concatenate/1
  Constant1/1 -> Vector Concatenate/2
  Multiply/1 -> Vector Concatenate/4
  Cos/1 -> Vector Concatenate/5
  Vector Concatenate/1 -> Selector2/1, Selector1/1, Selector/1
  Selector/1 -> Matrix Concatenate/1
  Selector1/1 -> Matrix Concatenate/2
  Selector2/1 -> Matrix Concatenate/3
  Matrix Concatenate/1 -> Display/1, A3theta/1

== system lab7task/DCM/3x3 Skew-symmetric matrix ==
  w : Inport
  Constant : Constant  Value=0
  Display : Display
  Matrix Concatenate : Concatenate  NumInputs=3  Mode=Multidimensional array  ConcatenateDimension=2
  Multiply : Gain  Gain=-1
  Scope : Scope
  Selector : Selector  InputPortWidth=7  IndexOptions=Index vector (dialog)  Indices=[4 1 5]  OutputSizes=1
  Selector1 : Selector  InputPortWidth=7  IndexOptions=Index vector (dialog)  Indices=[1 7 3]  OutputSizes=1
  Selector2 : Selector  InputPortWidth=7  IndexOptions=Index vector (dialog)  Indices=[6 2 1]  OutputSizes=1
  Transpose : Math  Operator=transpose
  Vector Concatenate : Concatenate  NumInputs=3
  w^ : Outport
  wires:
  Matrix Concatenate/1 -> Transpose/1
  Selector/1 -> Matrix Concatenate/2
  Selector2/1 -> Matrix Concatenate/3
  Selector1/1 -> Matrix Concatenate/1
  Vector Concatenate/1 -> Selector2/1, Selector/1, Selector1/1
  Constant/1 -> Vector Concatenate/1
  w/1 -> Scope/1, Multiply/1, Vector Concatenate/2
  Multiply/1 -> Vector Concatenate/3  "-w"
  Transpose/1 -> Display/1, w^/1

== system lab7task/Euler angles 312+313 /If Action Subsystem ==
  euler312 : Inport
  Action Port : ActionPort  ActionPortLabel=if(u1 > 0.1)
  A1rotation : Subsystem
  A2rotation : Subsystem
  A3rotation : Subsystem
  Demux : Demux  Outputs=3
  Display : Display
  Matrix Multiply : Product  Inputs=3  Multiplication=Matrix(*)
  A : Outport
  wires:
  euler312/1 -> Demux/1
  Matrix Multiply/1 -> Display/1, A/1
  A2rotation/1(matrix) -> Matrix Multiply/1
  A1rotation/1(matrix) -> Matrix Multiply/2
  A3rotation/1(matrix) -> Matrix Multiply/3
  Demux/1 -> A3rotation/1(angle)
  Demux/2 -> A1rotation/1(angle)
  Demux/3 -> A2rotation/1(angle)

== system lab7task/Euler angles 312+313 /If Action Subsystem1 ==
  euler313 : Inport
  Action Port : ActionPort  ActionPortLabel=else
  A1rotation : Subsystem
  A3rotation : Subsystem
  A3rotation1 : Subsystem
  Demux : Demux  Outputs=3
  Display : Display
  Matrix Multiply : Product  Inputs=3  Multiplication=Matrix(*)
  A : Outport
  wires:
  euler313/1 -> Demux/1
  A1rotation/1(matrix) -> Matrix Multiply/2
  A3rotation1/1(matrix) -> Matrix Multiply/1
  A3rotation/1(matrix) -> Matrix Multiply/3
  Matrix Multiply/1 -> A/1, Display/1
  Demux/1 -> A3rotation/1(angle)
  Demux/2 -> A1rotation/1(angle)
  Demux/3 -> A3rotation1/1(angle)

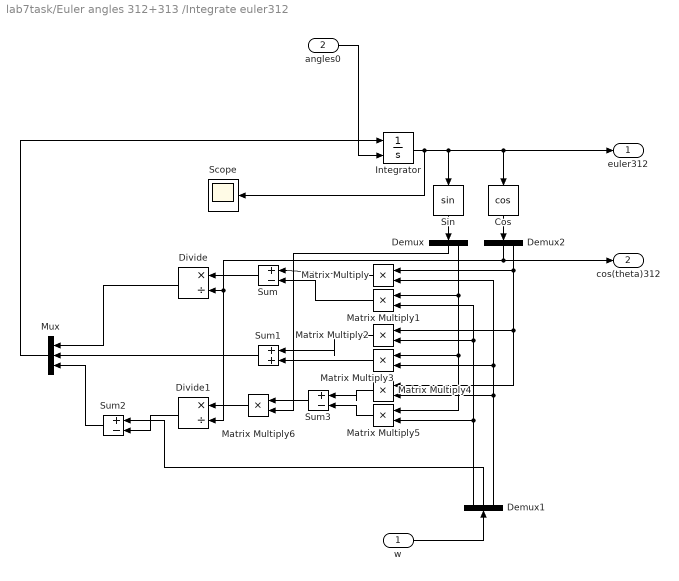
== system lab7task/Euler angles 312+313 /Integrate euler312 ==
  w : Inport
  angles0 : Inport  Port=2
  Cos : Trigonometry  Operator=cos
  Demux : Demux  Outputs=3
  Demux1 : Demux  Outputs=3
  Demux2 : Demux  Outputs=3
  Divide : Product  Inputs=*/
  Divide1 : Product  Inputs=*/
  Integrator : Integrator  InitialConditionSource=external
  Matrix Multiply{,1..6} (7 alike) : Product
  Mux : Mux  Inputs=3
  Scope : Scope
  Sin : Trigonometry
  Sum : Sum  Inputs=|+-
  Sum1 : Sum  Inputs=|++
  Sum2 : Sum  Inputs=|+-
  Sum3 : Sum  Inputs=|+-
  euler312 : Outport
  cos(theta)312 : Outport  Port=2
  wires:
  w/1 -> Demux1/1
  angles0/1 -> Integrator/2
  Integrator/1 -> Scope/1, Sin/1, Cos/1, euler312/1
  Mux/1 -> Integrator/1
  Sin/1 -> Demux/1
  Cos/1 -> Demux2/1
  Demux1/3 -> Matrix Multiply4/2, Matrix Multiply3/2, Matrix Multiply/2
  Demux2/3 -> Matrix Multiply4/1, Matrix Multiply2/1, Matrix Multiply/1
  Matrix Multiply/1 -> Sum/1
  Demux1/1 -> Matrix Multiply5/2, Matrix Multiply2/2, Matrix Multiply1/2
  Demux/3 -> Matrix Multiply5/1, Matrix Multiply3/1, Matrix Multiply1/1
  Matrix Multiply1/1 -> Sum/2
  Sum/1 -> Divide/1
  Divide/1 -> Mux/1
  Demux2/2 -> cos(theta)312/1, Divide1/2, Divide/2
  Matrix Multiply2/1 -> Sum1/1
  Matrix Multiply3/1 -> Sum1/2
  Sum1/1 -> Mux/2
  Sum2/1 -> Mux/3
  Matrix Multiply4/1 -> Sum3/1
  Matrix Multiply5/1 -> Sum3/2
  Sum3/1 -> Matrix Multiply6/1
  Demux/2 -> Matrix Multiply6/2
  Matrix Multiply6/1 -> Divide1/1
  Divide1/1 -> Sum2/2
  Demux1/2 -> Sum2/1

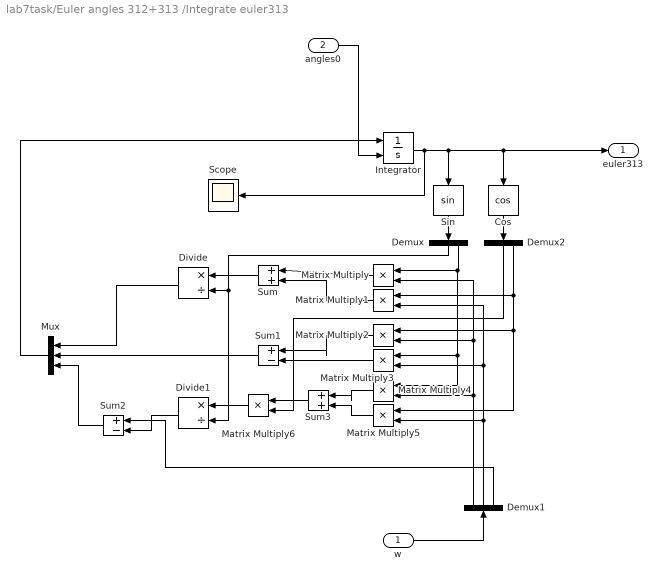
== system lab7task/Euler angles 312+313 /Integrate euler313 ==
  w : Inport
  angles0 : Inport  Port=2
  Cos : Trigonometry  Operator=cos
  Demux : Demux  Outputs=3
  Demux1 : Demux  Outputs=3
  Demux2 : Demux  Outputs=3
  Divide : Product  Inputs=*/
  Divide1 : Product  Inputs=*/
  Integrator : Integrator  InitialConditionSource=external
  Matrix Multiply{,1..6} (7 alike) : Product
  Mux : Mux  Inputs=3
  Scope : Scope
  Sin : Trigonometry
  Sum : Sum  Inputs=|++
  Sum1 : Sum  Inputs=|+-
  Sum2 : Sum  Inputs=|+-
  Sum3 : Sum  Inputs=|++
  euler313 : Outport
  wires:
  w/1 -> Demux1/1
  Cos/1 -> Demux2/1
  angles0/1 -> Integrator/2
  Sin/1 -> Demux/1
  Integrator/1 -> Scope/1, Sin/1, euler313/1, Cos/1
  Mux/1 -> Integrator/1
  Demux1/1 -> Matrix Multiply4/2, Matrix Multiply2/2, Matrix Multiply/2
  Matrix Multiply/1 -> Sum/1
  Matrix Multiply1/1 -> Sum/2
  Demux1/2 -> Matrix Multiply5/2, Matrix Multiply3/2, Matrix Multiply1/2
  Demux2/3 -> Matrix Multiply5/1, Matrix Multiply2/1, Matrix Multiply1/1
  Sum/1 -> Divide/1
  Demux/2 -> Divide1/2, Divide/2
  Divide/1 -> Mux/1
  Matrix Multiply2/1 -> Sum1/1
  Matrix Multiply3/1 -> Sum1/2
  Sum1/1 -> Mux/2
  Demux/3 -> Matrix Multiply4/1, Matrix Multiply3/1, Matrix Multiply/1
  Matrix Multiply4/1 -> Sum3/1
  Matrix Multiply5/1 -> Sum3/2
  Sum3/1 -> Matrix Multiply6/1
  Demux2/2 -> Matrix Multiply6/2
  Matrix Multiply6/1 -> Divide1/1
  Divide1/1 -> Sum2/2
  Demux1/3 -> Sum2/1
  Sum2/1 -> Mux/3

== system lab7task/Quaternion/4x4 Skew-symmetric matrix ==
  w : Inport
  Constant : Constant  Value=0
  Display : Display
  Matrix Concatenate : Concatenate  NumInputs=4  Mode=Multidimensional array  ConcatenateDimension=2
  Multiply : Gain  Gain=-1
  Selector : Selector  InputPortWidth=7  IndexOptions=Index vector (dialog)  Indices=[7 1 2 3]  OutputSizes=1
  Selector1 : Selector  InputPortWidth=7  IndexOptions=Index vector (dialog)  Indices=[1 4 6 2]  OutputSizes=1
  Selector2 : Selector  InputPortWidth=7  IndexOptions=Index vector (dialog)  Indices=[3 5 1 4]  OutputSizes=1
  Selector3 : Selector  InputPortWidth=7  IndexOptions=Index vector (dialog)  Indices=[5 6 7 1]  OutputSizes=1
  Transpose : Math  Operator=transpose
  Vector Concatenate : Concatenate  NumInputs=3
  w^ : Outport
  wires:
  Matrix Concatenate/1 -> Transpose/1
  Selector/1 -> Matrix Concatenate/2
  Selector2/1 -> Matrix Concatenate/3
  Selector1/1 -> Matrix Concatenate/1
  Vector Concatenate/1 -> Selector3/1, Selector2/1, Selector/1, Selector1/1
  Constant/1 -> Vector Concatenate/1
  w/1 -> Multiply/1, Vector Concatenate/2
  Multiply/1 -> Vector Concatenate/3  "-w"
  Selector3/1 -> Matrix Concatenate/4
  Transpose/1 -> Display/1, w^/1

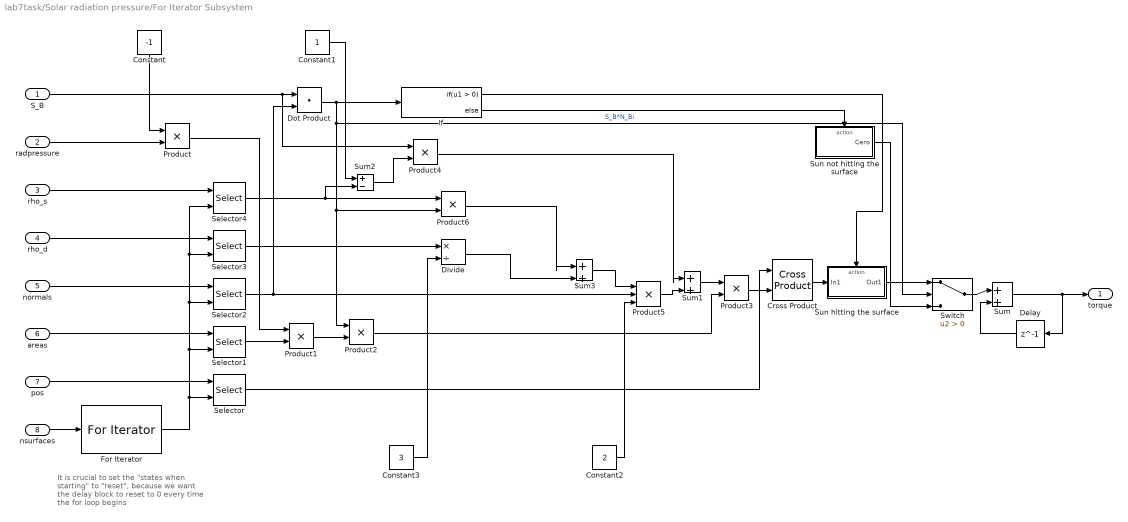
== system lab7task/Solar radiation pressure/For Iterator Subsystem ==
  note: It is crucial to set the "states when
      | starting" to "reset", because we want
      | the delay block to reset to 0 every
      | time the for loop begins
  S_B : Inport
  radpressure : Inport  Port=2
  rho_s : Inport  Port=3
  rho_d : Inport  Port=4
  normals : Inport  Port=5
  areas : Inport  Port=6
  pos : Inport  Port=7
  nsurfaces : Inport  Port=8
  Constant : Constant  Value=-1
  Constant1 : Constant
  Constant2 : Constant  Value=2
  Constant3 : Constant  Value=3
  Cross Product : matrix_library/Cross Product
  Delay : Delay  DelayLength=1
  Divide : Product  Inputs=*/
  Dot Product : DotProduct  OutDataTypeStr=Inherit: Inherit via internal rule
  For Iterator : ForIterator  ResetStates=reset  IterationSource=external
  If : If
  Product{,1..4,6} (6 alike) : Product
  Product5 : Product  Inputs=3
  Selector{,1..4} (5 alike) : Selector  NumberOfDimensions=2  InputPortWidth=3  IndexOptions=Select all,Index vector (port)  Indices=[1 3],1  OutputSizes=1,1
  Sum : Sum  Inputs=|++
  Sum1 : Sum  Inputs=|++
  Sum2 : Sum  Inputs=|+-
  Sum3 : Sum  Inputs=|++
  Sun hitting the surface : Subsystem  TreatAsAtomicUnit=on
  Sun not hitting the surface : Subsystem  TreatAsAtomicUnit=on
  Switch : Switch  Criteria=u2 > Threshold  SaturateOnIntegerOverflow=off  InputSameDT=off
  torque : Outport
  wires:
  nsurfaces/1 -> For Iterator/1
  Delay/1 -> Sum/2
  Sum/1 -> torque/1, Delay/1
  For Iterator/1 -> Selector1/2, Selector2/2, Selector3/2, Selector4/2, Selector/2
  pos/1 -> Selector/1
  rho_s/1 -> Selector4/1
  rho_d/1 -> Selector3/1
  normals/1 -> Selector2/1
  areas/1 -> Selector1/1
  S_B/1 -> Product4/1, Dot Product/1
  Selector2/1 -> Dot Product/2, Product5/2
  Dot Product/1 -> Switch/2, Product6/2, Product2/1, If/1  "S_B*N_Bi"
  Sun not hitting the surface/1(Cero) -> Switch/3
  If/1 -> Sun hitting the surface/Action
  If/2 -> Sun not hitting the surface/Action
  Switch/1 -> Sum/1
  Sun hitting the surface/1(Out1) -> Switch/1
  radpressure/1 -> Product/2
  Constant/1 -> Product/1
  Selector1/1 -> Product1/2
  Product/1 -> Product1/1
  Product1/1 -> Product2/2
  Cross Product/1 -> Sun hitting the surface/1(In1)
  Selector/1 -> Cross Product/1
  Product3/1 -> Cross Product/2
  Product2/1 -> Product3/2
  Sum1/1 -> Product3/1
  Constant1/1 -> Sum2/1
  Selector4/1 -> Product6/1, Sum2/2
  Sum2/1 -> Product4/2
  Product4/1 -> Sum1/1
  Product5/1 -> Sum1/2
  Sum3/1 -> Product5/1
  Constant2/1 -> Product5/3
  Product6/1 -> Sum3/1
  Selector3/1 -> Divide/1
  Divide/1 -> Sum3/2
  Constant3/1 -> Divide/2

== system lab7task/Air drag/For Iterator Subsystem/Air hitting the surface ==
  In1 : Inport
  Action Port : ActionPort  ActionPortLabel=if(u1 > 0)
  Out1 : Outport
  wires:
  In1/1 -> Out1/1

== system lab7task/Air drag/For Iterator Subsystem/Air not hitting the surface ==
  Action Port : ActionPort  ActionPortLabel=else
  Constant : Constant  Value=0
  Cero : Outport
  wires:
  Constant/1 -> Cero/1

== system lab7task/Euler angles 312+313 /If Action Subsystem/A1rotation ==
  angle : Inport
  Constant : Constant
  Constant1 : Constant  Value=0
  Cos : Trigonometry  Operator=cos
  Display : Display
  Matrix Concatenate : Concatenate  NumInputs=3  Mode=Multidimensional array  ConcatenateDimension=2
  Multiply : Gain  Gain=-1
  Selector : Selector  InputPortWidth=5  IndexOptions=Index vector (dialog)  Indices=[1 2 2]  OutputSizes=1
  Selector1 : Selector  InputPortWidth=5  IndexOptions=Index vector (dialog)  Indices=[2 5 4]  OutputSizes=1
  Selector2 : Selector  InputPortWidth=5  IndexOptions=Index vector (dialog)  Indices=[2 3 5]  OutputSizes=1
  Sin : Trigonometry
  Vector Concatenate : Concatenate  NumInputs=5
  matrix : Outport
  wires:
  angle/1 -> Cos/1, Sin/1
  Sin/1 -> Vector Concatenate/3, Multiply/1
  Constant/1 -> Vector Concatenate/1
  Constant1/1 -> Vector Concatenate/2
  Multiply/1 -> Vector Concatenate/4
  Cos/1 -> Vector Concatenate/5
  Vector Concatenate/1 -> Selector2/1, Selector1/1, Selector/1
  Selector/1 -> Matrix Concatenate/1
  Selector1/1 -> Matrix Concatenate/2
  Selector2/1 -> Matrix Concatenate/3
  Matrix Concatenate/1 -> Display/1, matrix/1

== system lab7task/Euler angles 312+313 /If Action Subsystem/A2rotation ==
  angle : Inport
  Constant : Constant
  Constant1 : Constant  Value=0
  Cos : Trigonometry  Operator=cos
  Display : Display
  Matrix Concatenate : Concatenate  NumInputs=3  Mode=Multidimensional array  ConcatenateDimension=2
  Multiply : Gain  Gain=-1
  Selector : Selector  InputPortWidth=5  IndexOptions=Index vector (dialog)  Indices=[5 2 3]  OutputSizes=1
  Selector1 : Selector  InputPortWidth=5  IndexOptions=Index vector (dialog)  Indices=[2 1 2]  OutputSizes=1
  Selector2 : Selector  InputPortWidth=5  IndexOptions=Index vector (dialog)  Indices=[4 2 5]  OutputSizes=1
  Sin : Trigonometry
  Vector Concatenate : Concatenate  NumInputs=5
  matrix : Outport
  wires:
  angle/1 -> Cos/1, Sin/1
  Sin/1 -> Vector Concatenate/3, Multiply/1
  Constant/1 -> Vector Concatenate/1
  Constant1/1 -> Vector Concatenate/2
  Multiply/1 -> Vector Concatenate/4
  Cos/1 -> Vector Concatenate/5
  Vector Concatenate/1 -> Selector2/1, Selector1/1, Selector/1
  Selector/1 -> Matrix Concatenate/1
  Selector1/1 -> Matrix Concatenate/2
  Selector2/1 -> Matrix Concatenate/3
  Matrix Concatenate/1 -> Display/1, matrix/1

== system lab7task/Euler angles 312+313 /If Action Subsystem/A3rotation ==
  angle : Inport
  Constant : Constant
  Constant1 : Constant  Value=0
  Cos : Trigonometry  Operator=cos
  Display : Display
  Matrix Concatenate : Concatenate  NumInputs=3  Mode=Multidimensional array  ConcatenateDimension=2
  Multiply : Gain  Gain=-1
  Selector : Selector  InputPortWidth=5  IndexOptions=Index vector (dialog)  Indices=[5 4 2]  OutputSizes=1
  Selector1 : Selector  InputPortWidth=5  IndexOptions=Index vector (dialog)  Indices=[3 5 2]  OutputSizes=1
  Selector2 : Selector  InputPortWidth=5  IndexOptions=Index vector (dialog)  Indices=[2 2 1]  OutputSizes=1
  Sin : Trigonometry
  Vector Concatenate : Concatenate  NumInputs=5
  matrix : Outport
  wires:
  angle/1 -> Cos/1, Sin/1
  Sin/1 -> Vector Concatenate/3, Multiply/1
  Constant/1 -> Vector Concatenate/1
  Constant1/1 -> Vector Concatenate/2
  Multiply/1 -> Vector Concatenate/4
  Cos/1 -> Vector Concatenate/5
  Vector Concatenate/1 -> Selector2/1, Selector1/1, Selector/1
  Selector/1 -> Matrix Concatenate/1
  Selector1/1 -> Matrix Concatenate/2
  Selector2/1 -> Matrix Concatenate/3
  Matrix Concatenate/1 -> Display/1, matrix/1

== system lab7task/Euler angles 312+313 /If Action Subsystem1/A1rotation ==
  angle : Inport
  Constant : Constant
  Constant1 : Constant  Value=0
  Cos : Trigonometry  Operator=cos
  Display : Display
  Matrix Concatenate : Concatenate  NumInputs=3  Mode=Multidimensional array  ConcatenateDimension=2
  Multiply : Gain  Gain=-1
  Selector : Selector  InputPortWidth=5  IndexOptions=Index vector (dialog)  Indices=[1 2 2]  OutputSizes=1
  Selector1 : Selector  InputPortWidth=5  IndexOptions=Index vector (dialog)  Indices=[2 5 4]  OutputSizes=1
  Selector2 : Selector  InputPortWidth=5  IndexOptions=Index vector (dialog)  Indices=[2 3 5]  OutputSizes=1
  Sin : Trigonometry
  Vector Concatenate : Concatenate  NumInputs=5
  matrix : Outport
  wires:
  angle/1 -> Cos/1, Sin/1
  Sin/1 -> Vector Concatenate/3, Multiply/1
  Constant/1 -> Vector Concatenate/1
  Constant1/1 -> Vector Concatenate/2
  Multiply/1 -> Vector Concatenate/4
  Cos/1 -> Vector Concatenate/5
  Vector Concatenate/1 -> Selector2/1, Selector1/1, Selector/1
  Selector/1 -> Matrix Concatenate/1
  Selector1/1 -> Matrix Concatenate/2
  Selector2/1 -> Matrix Concatenate/3
  Matrix Concatenate/1 -> Display/1, matrix/1

== system lab7task/Euler angles 312+313 /If Action Subsystem1/A3rotation ==
  angle : Inport
  Constant : Constant
  Constant1 : Constant  Value=0
  Cos : Trigonometry  Operator=cos
  Display : Display
  Matrix Concatenate : Concatenate  NumInputs=3  Mode=Multidimensional array  ConcatenateDimension=2
  Multiply : Gain  Gain=-1
  Selector : Selector  InputPortWidth=5  IndexOptions=Index vector (dialog)  Indices=[5 4 2]  OutputSizes=1
  Selector1 : Selector  InputPortWidth=5  IndexOptions=Index vector (dialog)  Indices=[3 5 2]  OutputSizes=1
  Selector2 : Selector  InputPortWidth=5  IndexOptions=Index vector (dialog)  Indices=[2 2 1]  OutputSizes=1
  Sin : Trigonometry
  Vector Concatenate : Concatenate  NumInputs=5
  matrix : Outport
  wires:
  angle/1 -> Cos/1, Sin/1
  Sin/1 -> Vector Concatenate/3, Multiply/1
  Constant/1 -> Vector Concatenate/1
  Constant1/1 -> Vector Concatenate/2
  Multiply/1 -> Vector Concatenate/4
  Cos/1 -> Vector Concatenate/5
  Vector Concatenate/1 -> Selector2/1, Selector1/1, Selector/1
  Selector/1 -> Matrix Concatenate/1
  Selector1/1 -> Matrix Concatenate/2
  Selector2/1 -> Matrix Concatenate/3
  Matrix Concatenate/1 -> Display/1, matrix/1

== system lab7task/Euler angles 312+313 /If Action Subsystem1/A3rotation1 ==
  angle : Inport
  Constant : Constant
  Constant1 : Constant  Value=0
  Cos : Trigonometry  Operator=cos
  Display : Display
  Matrix Concatenate : Concatenate  NumInputs=3  Mode=Multidimensional array  ConcatenateDimension=2
  Multiply : Gain  Gain=-1
  Selector : Selector  InputPortWidth=5  IndexOptions=Index vector (dialog)  Indices=[5 4 2]  OutputSizes=1
  Selector1 : Selector  InputPortWidth=5  IndexOptions=Index vector (dialog)  Indices=[3 5 2]  OutputSizes=1
  Selector2 : Selector  InputPortWidth=5  IndexOptions=Index vector (dialog)  Indices=[2 2 1]  OutputSizes=1
  Sin : Trigonometry
  Vector Concatenate : Concatenate  NumInputs=5
  matrix : Outport
  wires:
  angle/1 -> Cos/1, Sin/1
  Sin/1 -> Vector Concatenate/3, Multiply/1
  Constant/1 -> Vector Concatenate/1
  Constant1/1 -> Vector Concatenate/2
  Multiply/1 -> Vector Concatenate/4
  Cos/1 -> Vector Concatenate/5
  Vector Concatenate/1 -> Selector2/1, Selector1/1, Selector/1
  Selector/1 -> Matrix Concatenate/1
  Selector1/1 -> Matrix Concatenate/2
  Selector2/1 -> Matrix Concatenate/3
  Matrix Concatenate/1 -> Display/1, matrix/1

== system lab7task/Solar radiation pressure/For Iterator Subsystem/Sun hitting the surface ==
  In1 : Inport
  Action Port : ActionPort  ActionPortLabel=if(u1 > 0)
  Out1 : Outport
  wires:
  In1/1 -> Out1/1

== system lab7task/Solar radiation pressure/For Iterator Subsystem/Sun not hitting the surface ==
  Action Port : ActionPort  ActionPortLabel=else
  Constant : Constant  Value=0
  Cero : Outport
  wires:
  Constant/1 -> Cero/1
